simulink model "ctrl_stab_new"  (R2014b)
settings: Solver=ode45  StartTime=0.0  StopTime=10  FixedStep=0.01  MaxStep=1e-3  MinStep=1e-5  RelTol=1e-3
PreLoadFcn:
  | load('imu');
undefined symbols (not defined in the file or in its folder): Tp2p
libraries: simulink x2, slident x1, dspsrcs4 x1
settings Model: Creator=Ugo Pattacini  LastModifiedBy=Ugo Pattacini
settings DataIOCC: LimitDataPoints=off  SaveOutput=off  SaveTime=off
settings DebuggingCC: UnderspecifiedInitializationDetection=Classic  MergeDetectMultiDrivingBlocksExec=none

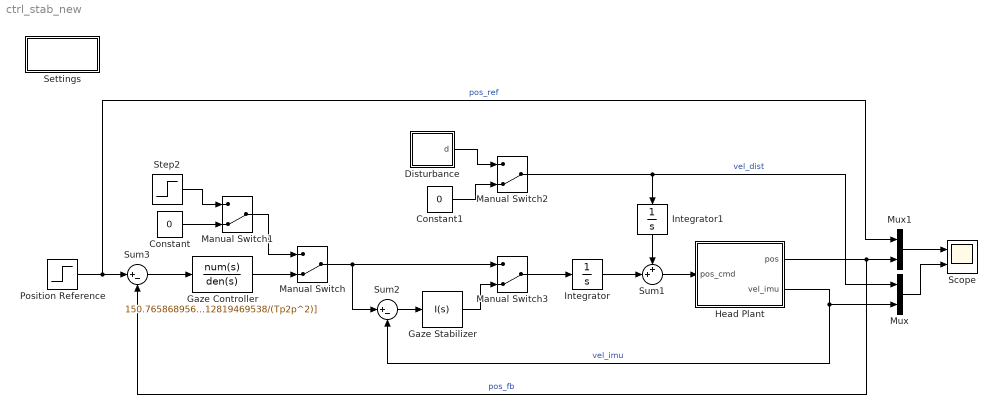
== system ctrl_stab_new ==
  Constant : Constant  Value=0
  Constant1 : Constant  Value=0
  Disturbance : Subsystem  mask{t0=1.2, T=3, A=-20}
      mask prompts: t0 "Start Time [s]"; T "Duration [s]"; A "Amplitude"
      mask help: Settings for Disturbance Model
  Gaze Controller : TransferFcn  Numerator=150.765868956161/(Tp2p^3)  Denominator=[1 15.9669610709384/Tp2p 84.9812819469538/(Tp2p^2)]
  Gaze Stabilizer : simulink/Continuous/PID Controller  Controller=I  TimeDomain=Continuous-time  SampleTime=-1  IntegratorMethod=Trapezoidal  FilterMethod=Trapezoidal  Form=Parallel  P=0  I=11  D=0  N=100  InitialConditionSource=internal  InitialConditionForIntegrator=0  InitialConditionForFilter=0  ExternalReset=none  LimitOutput=off  UpperSaturationLimit=inf  LowerSaturationLimit=-inf  LinearizeAsGain=off  AntiWindupMode=none  Kb=1  TrackingMode=off  Kt=1  PParamMin=[]  PParamMax=[]  IParamMin=[]  IParamMax=[]  DParamMin=[]  DParamMax=[]  NParamMin=[]  NParamMax=[]  KbParamMin=[]  KbParamMax=[]  KtParamMin=[]  KtParamMax=[]  POutMin=[]  POutMax=[]  IOutMin=[]  IOutMax=[]  DOutMin=[]  DOutMax=[]  NOutMin=[]  NOutMax=[]  KbOutMin=[]  KbOutMax=[]  KtOutMin=[]  KtOutMax=[]  IntegratorOutMin=[]  IntegratorOutMax=[]  FilterOutMin=[]  FilterOutMax=[]  SumOutMin=[]  SumOutMax=[]  SumI1OutMin=[]  SumI1OutMax=[]  SumI2OutMin=[]  SumI2OutMax=[]  SumI3OutMin=[]  SumI3OutMax=[]  SumDOutMin=[]  SumDOutMax=[]  SaturationOutMin=[]  SaturationOutMax=[]  IntegratorContinuousStateAttributes=''  IntegratorStateMustResolveToSignalObject=off  IntegratorRTWStateStorageClass=Auto  FilterContinuousStateAttributes=''  FilterStateMustResolveToSignalObject=off  FilterRTWStateStorageClass=Auto  DifferentiatorICPrevScaledInput=0  DifferentiatorOutMin=[]  DifferentiatorOutMax=[]  UseFilter=on
  Head Plant : Subsystem
  Integrator : Integrator
  Integrator1 : Integrator
  Manual Switch{,1..3} (4 alike) : ManualSwitch  CurrentSetting=0
  Mux : Mux  Inputs=2
  Mux1 : Mux  Inputs=2
  Position Reference : Step  After=10  SampleTime=0
  Scope : Scope  NumInputPorts=2
      settings: ShowLegends=on  TimeRange=10  YMin=-2~-20  YMax=12~40
  Settings : Subsystem  mask{Tp2p=0.5}
      mask prompts: Tp2p "Controller point-to-point trajectory time [s]"
      mask help: Model Settings
      mask init:
      | assignin('base','Tp2p',Tp2p);
      mask Display: disp(sprintf('Tp2p = %g',Tp2p));
  Step2 : Step  Time=2  After=30  SampleTime=0
  Sum1 : Sum  Inputs=++|
  Sum2 : Sum  Inputs=|+-
  Sum3 : Sum  Inputs=|+-
  wires:
  Sum1/1 -> Head Plant/1(pos_cmd)
  Sum2/1 -> Gaze Stabilizer/1
  Head Plant/2(vel_imu) -> Sum2/2, Mux/2  "vel_imu"
  Manual Switch/1 -> Manual Switch3/1, Sum2/1
  Gaze Controller/1 -> Manual Switch/2
  Sum3/1 -> Gaze Controller/1
  Head Plant/1(pos) -> Mux1/2, Sum3/2  "pos_fb"
  Manual Switch1/1 -> Manual Switch/1
  Constant/1 -> Manual Switch1/2
  Step2/1 -> Manual Switch1/1
  Mux/1 -> Scope/2
  Mux1/1 -> Scope/1
  Position Reference/1 -> Mux1/1, Sum3/1  "pos_ref"
  Constant1/1 -> Manual Switch2/2
  Disturbance/1(d) -> Manual Switch2/1
  Manual Switch2/1 -> Mux/1, Integrator1/1  "vel_dist"
  Gaze Stabilizer/1 -> Manual Switch3/2
  Manual Switch3/1 -> Integrator/1
  Integrator/1 -> Sum1/2
  Integrator1/1 -> Sum1/1

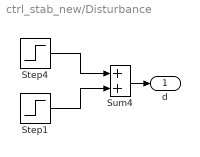
== system ctrl_stab_new/Disturbance ==
  Step1 : Step  Time=t0+T  After=-A  SampleTime=0
  Step4 : Step  Time=t0  After=A  SampleTime=0
  Sum4 : Sum
  d : Outport
  wires:
  Sum4/1 -> d/1
  Step4/1 -> Sum4/1
  Step1/1 -> Sum4/2

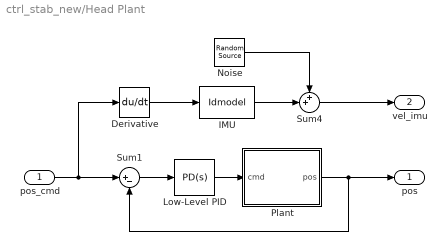
== system ctrl_stab_new/Head Plant ==
  pos_cmd : Inport
  Derivative : Derivative
  "IMU " : slident/Models/Idmodel  sys=imu  IC=0  noi=off  seed=[]
  Low-Level PID : simulink/Continuous/PID Controller  Controller=PD  TimeDomain=Continuous-time  SampleTime=-1  IntegratorMethod=Trapezoidal  FilterMethod=Trapezoidal  Form=Parallel  P=122.195125158059  I=1  D=53.9650314282148  N=94.0864796738016  InitialConditionSource=internal  InitialConditionForIntegrator=0  InitialConditionForFilter=0  ExternalReset=none  LimitOutput=off  UpperSaturationLimit=inf  LowerSaturationLimit=-inf  LinearizeAsGain=off  AntiWindupMode=none  Kb=1  TrackingMode=off  Kt=1  PParamMin=[]  PParamMax=[]  IParamMin=[]  IParamMax=[]  DParamMin=[]  DParamMax=[]  NParamMin=[]  NParamMax=[]  KbParamMin=[]  KbParamMax=[]  KtParamMin=[]  KtParamMax=[]  POutMin=[]  POutMax=[]  IOutMin=[]  IOutMax=[]  DOutMin=[]  DOutMax=[]  NOutMin=[]  NOutMax=[]  KbOutMin=[]  KbOutMax=[]  KtOutMin=[]  KtOutMax=[]  IntegratorOutMin=[]  IntegratorOutMax=[]  FilterOutMin=[]  FilterOutMax=[]  SumOutMin=[]  SumOutMax=[]  SumI1OutMin=[]  SumI1OutMax=[]  SumI2OutMin=[]  SumI2OutMax=[]  SumI3OutMin=[]  SumI3OutMax=[]  SumDOutMin=[]  SumDOutMax=[]  SaturationOutMin=[]  SaturationOutMax=[]  IntegratorContinuousStateAttributes=''  IntegratorStateMustResolveToSignalObject=off  IntegratorRTWStateStorageClass=Auto  FilterContinuousStateAttributes=''  FilterStateMustResolveToSignalObject=off  FilterRTWStateStorageClass=Auto  DifferentiatorICPrevScaledInput=0  DifferentiatorOutMin=[]  DifferentiatorOutMax=[]  UseFilter=on
  Noise : dspsrcs4/Random Source  SrcType=Gaussian  NormMethod=Ziggurat  CltLength=12  MinVal=0  MaxVal=1  MeanVal=0  VarVal=0.2  RepMode=Not repeatable  rawSeed=1  IsInherit=off  SampMode=Continuous  SampTime=1  SampFrame=1  DataType=Double  OutComplex=Real
  Plant : Subsystem
  Sum1 : Sum  Inputs=|+-
  Sum4 : Sum  Inputs=++|
  pos : Outport
  vel_imu : Outport  Port=2
  wires:
  Low-Level PID/1 -> Plant/1(cmd)
  Sum1/1 -> Low-Level PID/1
  Plant/1(pos) -> Sum1/2, pos/1
  pos_cmd/1 -> Sum1/1, Derivative/1
  "IMU "/1 -> Sum4/2
  Sum4/1 -> vel_imu/1
  Noise/1 -> Sum4/1
  Derivative/1 -> "IMU "/1

== system ctrl_stab_new/Settings ==

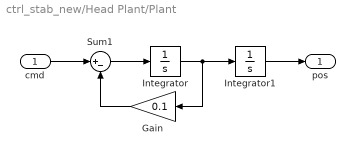
== system ctrl_stab_new/Head Plant/Plant ==
  cmd : Inport
  Gain : Gain  Gain=0.1
  Integrator : Integrator
  Integrator1 : Integrator
  Sum1 : Sum  Inputs=|+-
  pos : Outport
  wires:
  Integrator/1 -> Gain/1, Integrator1/1
  Sum1/1 -> Integrator/1
  Integrator1/1 -> pos/1
  cmd/1 -> Sum1/1
  Gain/1 -> Sum1/2
